simulink model "pruebaSF3_truetime"  (R2018a)
settings: Solver=FixedStepAuto  StartTime=0.0  StopTime=6  FixedStep=0.0001  RelTol=1e-3
InitFcn:
  | SimulinkInit
values from neighbouring files (symbols this model uses):
  C = C1+C2+C3+Cl    (= 0.002654)    [SimulinkInit.m]
  C3 = 610e-6    (= 0.00061)    [SimulinkInit.m]
  J = 0.3    [SimulinkInit.m]
  K1 = 1.15    [SimulinkInit.m]
  K2 = 1    [SimulinkInit.m]
  K3 = 1    [SimulinkInit.m]
  L1 = 40e-3    (= 0.04)    [SimulinkInit.m]
  L2 = 5e-3    (= 0.005)    [SimulinkInit.m]
  L3 = 30e-3    (= 0.03)    [SimulinkInit.m]
  L4 = 5.2    [SimulinkInit.m]
  P = 0.1    [SimulinkInit.m]
  R1 = 0.1    [SimulinkInit.m]
  R2 = 0.1    [SimulinkInit.m]
  R3 = 1e-3    (= 0.001)    [SimulinkInit.m]
  R4 = 10    [SimulinkInit.m]
  R5 = 10    [SimulinkInit.m]
  Tao1 = 0.5    [SimulinkInit.m]
  Tao2 = 0.125    [SimulinkInit.m]
libraries: dsparch4 x5, truetime x2, mpclib x2, simulink x1, powerlib_meascontrol x1
settings Model: Creator=carma  LastModifiedBy=carma
settings CodeAppCC: StateflowObjectComments=on
settings SimscapeCC: SimscapeNormalizeSystem=off

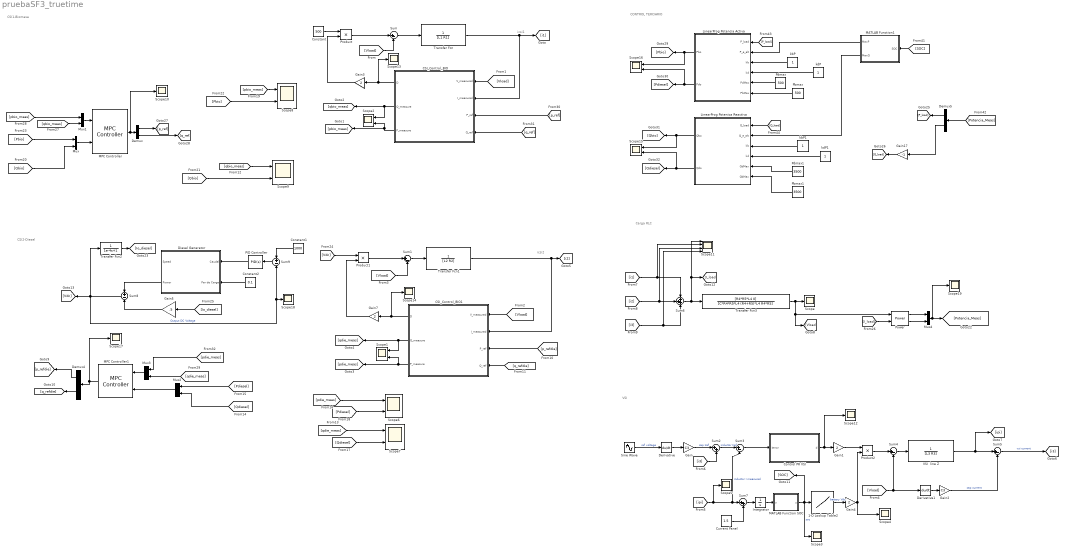
== system pruebaSF3_truetime ==
  note: Carga RLC
  note: CONTROL TERCIARIO
  note: CSI1-Biomasa
  note: CSI2-Diesel
  note: VSI
  note: icsi2
  note: icsi1
  1-D Lookup Table2 : Lookup_n-D  NumberOfTableDimensions=1  BreakpointsForDimension1=[0 10 20 30 40 50 70 80 100]  Table=[0 10 200 500 800 1000 1140 1150 1200]  InternalRulePriority=Speed  RndMeth=Simplest  InputSameDT=on
  CSI_Control_BIO : Subsystem  mask{A=[0.0201   -0.039932     0.01986], B=[1     -1.9966       0.998], T=0.0001, st_time=.1, Dn=[1     -1.0364], Dd=[1    -0.96364]}
      mask prompts: A "Numerador del control PR(z)"; B "Denominador del control PR(z)"; T "Tiempo de muestreo"; st_time "Tiempo_muerto"; Dn "Dn (Numerador de D(z))"; Dd "Dd (numerador de D(z))"
      mask DialogControl descripcion Prompt: Lazo de control de corriente para inversor monofasico. La entrada es un setpoint de potencia [P, Q]. Con ese setpoint se calcula la referencia de corriente sinusoidal deacuerdo a la tension medida de la red. Por lo anterior este controlador solo es valido para un inversor conectado a la red pues hara que se comporte como un CSI.
      mask DialogControl Control2 Prompt: Dn y Dd corresponden al numerador y denominador de la funcion de transferencia en Z (denominada D(z)) que hara un desfase de 90 de las señales medidas de tension y corriente del inversor. Estos desfases permiten mimificar las señales alfa y beta, de esta forma usar la misma teoria de potencia instantanea para el caso monofasico.
  CSI_Control_BIO1 : Subsystem  mask{A=[0.0201   -0.039932     0.01986], B=[1     -1.9966       0.998], T=0.0001, st_time=.1, Dn=[1     -1.0364], Dd=[1    -0.96364]}
      mask prompts: A "Numerador del control PR(z)"; B "Denominador del control PR(z)"; T "Tiempo de muestreo"; st_time "Tiempo_muerto"; Dn "Dn (Numerador de D(z))"; Dd "Dd (numerador de D(z))"
      mask DialogControl descripcion Prompt: Lazo de control de corriente para inversor monofasico. La entrada es un setpoint de potencia [P, Q]. Con ese setpoint se calcula la referencia de corriente sinusoidal deacuerdo a la tension medida de la red. Por lo anterior este controlador solo es valido para un inversor conectado a la red pues hara que se comporte como un CSI.
      mask DialogControl Control2 Prompt: Dn y Dd corresponden al numerador y denominador de la funcion de transferencia en Z (denominada D(z)) que hara un desfase de 90 de las señales medidas de tension y corriente del inversor. Estos desfases permiten mimificar las señales alfa y beta, de esta forma usar la misma teoria de potencia instantanea para el caso monofasico.
  Constant : Constant  Value=500
  Constant1 : Constant  Value=1000
  Constant2 : Constant  Value=0.1
  Control PR VSI : Subsystem
  Current Panel : Constant  Value=1.5
  Demux : Demux  Outputs=2
  Demux4 : Demux  Outputs=2
  Demux5 : Demux  Outputs=2
  Derivative : Derivative
  Derivative1 : Derivative
  Diesel Generator : Subsystem
  Gain : Gain  Gain=C3
  Gain{1,3..4,7} (4 alike) : Gain  Gain=2
  Gain17 : Gain  Gain=-1
  Gain2 : Gain  Gain=C3
  Gain5 : Gain  Gain=.5
  Integrator : Integrator  LimitOutput=on  UpperSaturationLimit=1  LowerSaturationLimit=0
  LinearProg Potencia Activa : MATLAB Function  TreatAsAtomicUnit=on  SystemSampleTime=.03
  LinearProg Potenica Reactiva : MATLAB Function  TreatAsAtomicUnit=on  SystemSampleTime=.03
  "MATLAB Function SOC " : MATLAB Function  TreatAsAtomicUnit=on
  MATLAB Function1 : MATLAB Function  TreatAsAtomicUnit=on
  MPC Controller : mpclib/MPC Controller  mpcobj=mpcobj  x0=[]  is_multiple=0  enable_value=0  return_u0=off  updateMPCinCallerWorkspace=on  ref_from_ws=off  ref_signal_name=[]  ref_preview=on  md_from_ws=off  md_signal_name=[]  md_preview=on  from_project=off  project_file=MPCtask.mat  md_inport=off  mv_inport=off  cost_outport=off  return_sequence=off  return_qpstatus=off  return_state=off  state_inport=off  lims_inport=off  cc_inport=off  ywt_inport=off  is_designfromscratch=0  uwt_inport=off  duwt_inport=off  rhoeps_inport=off  uref_inport=off  n_ts=0.1  n_p=100  n_mv=2  n_md=0  n_ud=0  n_mo=2  n_uo=0  BlockDataType=double  SampleTimeInherited=off  switch_inport=off
  MPC Controller1 : mpclib/MPC Controller  mpcobj=mpcobj  x0=[]  is_multiple=0  enable_value=0  return_u0=off  updateMPCinCallerWorkspace=on  ref_from_ws=off  ref_signal_name=[]  ref_preview=on  md_from_ws=off  md_signal_name=[]  md_preview=on  from_project=off  project_file=MPCtask.mat  md_inport=off  mv_inport=off  cost_outport=off  return_sequence=off  return_qpstatus=off  return_state=off  state_inport=off  lims_inport=off  cc_inport=off  ywt_inport=off  is_designfromscratch=0  uwt_inport=off  duwt_inport=off  rhoeps_inport=off  uref_inport=off  n_ts=0.1  n_p=100  n_mv=2  n_md=0  n_ud=0  n_mo=2  n_uo=0  BlockDataType=double  SampleTimeInherited=off  switch_inport=off
  Mux{,1..4} (5 alike) : Mux  Inputs=2
  PID Controller : simulink/Continuous/PID Controller  Controller=PID  TimeDomain=Continuous-time  SampleTime=-1  IntegratorMethod=Forward Euler  FilterMethod=Forward Euler  Form=Parallel  UseFilter=on  ControllerParametersSource=internal  P=0.000853612192208084  I=3.94394231511782e-05  D=0.00224356290205903  N=0.155980576752107  InitialConditionSource=internal  InitialConditionForIntegrator=0  InitialConditionForFilter=0  ExternalReset=none  LimitOutput=off  UpperSaturationLimit=inf  LowerSaturationLimit=-inf  LinearizeAsGain=on  AntiWindupMode=none  Kb=1  TrackingMode=off  Kt=1  PParamMin=[]  PParamMax=[]  IParamMin=[]  IParamMax=[]  DParamMin=[]  DParamMax=[]  NParamMin=[]  NParamMax=[]  KbParamMin=[]  KbParamMax=[]  KtParamMin=[]  KtParamMax=[]  POutMin=[]  POutMax=[]  IOutMin=[]  IOutMax=[]  DOutMin=[]  DOutMax=[]  NOutMin=[]  NOutMax=[]  KbOutMin=[]  KbOutMax=[]  KtOutMin=[]  KtOutMax=[]  IntegratorOutMin=[]  IntegratorOutMax=[]  FilterOutMin=[]  FilterOutMax=[]  SumOutMin=[]  SumOutMax=[]  SumI1OutMin=[]  SumI1OutMax=[]  SumI2OutMin=[]  SumI2OutMax=[]  SumI3OutMin=[]  SumI3OutMax=[]  SumDOutMin=[]  SumDOutMax=[]  SaturationOutMin=[]  SaturationOutMax=[]  IntegratorContinuousStateAttributes=''  IntegratorStateMustResolveToSignalObject=off  IntegratorRTWStateStorageClass=Auto  FilterContinuousStateAttributes=''  FilterStateMustResolveToSignalObject=off  FilterRTWStateStorageClass=Auto  DifferentiatorICPrevScaledInput=0  DifferentiatorOutMin=[]  DifferentiatorOutMax=[]  InitialConditionSetting=State (most efficient)  FilterDiffOutCoefMin=[]  FilterDiffOutCoefMax=[]  SumDenOutMin=[]  SumDenOutMax=[]  SumNumOutMin=[]  SumNumOutMax=[]  ReciprocalOutMin=[]  ReciprocalOutMax=[]  DivideOutMin=[]  DivideOutMax=[]  TunerSelectOption=Transfer Function Based (PID Tuner App)
  Pbmax : Constant  Value=500
  Pbmax1 : Constant  Value=3500
  Pdmax : Constant  Value=500
  Pdmax1 : Constant  Value=3500
  Power : powerlib_meascontrol/Measurements/Power  Freq=60  Vinit=[1, 0]  Iinit=[1, 0]  Ts=0
      settings: SourceProductName=Simscape Power Systems
  Product : Product
  Product1 : Product
  Product2 : Product
  Scope{,3..5,10,12..14,17..19} (11 alike) : Scope
  Scope{1..2,6..9,15..16} (8 alike) : Scope  NumInputPorts=2
  Scope11 : Scope  NumInputPorts=4
  Sine Wave : Sin  Amplitude=170  Frequency=2*pi*60  SampleTime=0
  Sum{,1,3..5} (5 alike) : Sum  Inputs=|+-
  Sum2 : Sum  Inputs=|++
  Sum6 : Sum  Inputs=3
  Sum7 : Sum  Inputs=|++
  Sum8 : Sum  Inputs=+-
  Sum9 : Sum  Inputs=+-
  Transfer Fcn : TransferFcn  Denominator=[L1 R1]
  Transfer Fcn1 : TransferFcn  Denominator=[L2 R2]
  Transfer Fcn2 : TransferFcn  Denominator=[1e-4 1]
  Transfer Fcn3 : TransferFcn  Numerator=[R4*R5*L4 0]  Denominator=[C*R4*R5*L4 (R4+R5)*L4 R4*R5]
  VSI  line Z : TransferFcn  Denominator=[L3 R3]
  kbP : Constant
  kbP1 : Constant
  kdP : Constant
  kdP1 : Constant
  wires:
  Sum/1 -> Transfer Fcn/1
  [Vload] -> Sum/2
  Product/1 -> Sum/1
  Constant/1 -> Product/1
  Gain3/1 -> Product/2
  CSI_Control_BIO/2(Q_measure) -> [qbio_meas], Scope2/1
  Transfer Fcn/1 -> [i1], CSI_Control_BIO/2(I_measured)
  [Vload] -> CSI_Control_BIO/1(V_measured)
  CSI_Control_BIO/1(D) -> Scope13/1, Gain3/1
  Gain7/1 -> Product1/2
  CSI_Control_BIO1/1(D) -> Scope14/1, Gain7/1
  Transfer Fcn1/1 -> [i2], CSI_Control_BIO1/2(I_measured)
  [Vload] -> CSI_Control_BIO1/1(V_measured)
  CSI_Control_BIO1/3(P_measure) -> Scope1/2, [pdie_meas]
  CSI_Control_BIO1/2(Q_measure) -> [qdie_meas], Scope1/1
  Product1/1 -> Sum1/1
  [Vdc] -> Product1/1
  Sum1/1 -> Transfer Fcn1/1
  [Vload] -> Sum1/2
  Sine Wave/1 -> Derivative/1  "ref voltage"
  Derivative/1 -> Gain/1
  Gain/1 -> Sum2/1  "cap Iref"
  Sum2/1 -> Sum3/1  "inductor Iref"
  Sum3/1 -> Control PR VSI/1(Ierror)
  Control PR VSI/1(d) -> Scope12/1, Gain1/1
  Gain1/1 -> Product2/1
  Product2/1 -> Sum4/1
  [Vload] -> Sum4/2, Derivative1/1
  Derivative1/1 -> Gain2/1
  Sum4/1 -> VSI  line Z/1
  VSI  line Z/1 -> [ipi], Sum5/1
  Gain2/1 -> Sum5/2  "cap current"
  Sum5/1 -> [i3]  "vsi current"
  [ipi] -> Scope5/1, Sum7/1, Sum3/2  "inductor I measured"
  [i3] -> Sum2/2
  Integrator/1 -> "MATLAB Function SOC "/1(u)
  "MATLAB Function SOC "/1(y) -> [SOC], Scope3/1, 1-D Lookup Table2/1  "soc"
  1-D Lookup Table2/1 -> Gain4/1  "battery Vdc"
  [i1] -> Scope11/2, Sum6/1
  [i2] -> Scope11/3, Sum6/2
  [i3] -> Sum6/3, Scope11/4
  Sum6/1 -> [I_load], Scope11/1, Transfer Fcn3/1
  [qdie_meas] -> Scope7/1
  Mux3/1 -> MPC Controller1/1
  [pdie_meas] -> Mux3/1
  Demux4/2 -> [q_refdie]
  Mux2/1 -> MPC Controller1/2
  [qdie_meas] -> Mux3/2
  [Qdiesel] -> Scope7/2
  MPC Controller1/1 -> Demux4/1, Scope17/1
  [Pdiesel] -> Scope6/2
  [pdie_meas] -> Scope6/1
  Demux4/1 -> [p_refdie]
  [pbio_meas] -> Mux1/1
  [Pbio] -> Scope8/2
  [qbio_meas] -> Scope9/1
  [qbio_meas] -> Mux1/2
  MPC Controller/1 -> Scope10/1, Demux/1
  [Qbio] -> Scope9/2
  Mux1/1 -> MPC Controller/1
  Demux/2 -> [q_ref]
  [pbio_meas] -> Scope8/1
  Mux/1 -> MPC Controller/2
  Demux/1 -> [p_ref]
  [SOC] -> MATLAB Function1/1(SOC)
  kdP/1 -> LinearProg Potencia Activa/4(kd)
  Pdmax/1 -> LinearProg Potencia Activa/5(PdMax)
  Gain17/1 -> [Q_load]
  kbP1/1 -> LinearProg Potenica Reactiva/3(kb)
  LinearProg Potencia Activa/2(Pdo) -> Scope16/2, [Pdiesel]
  [P_load] -> LinearProg Potencia Activa/1(P_load)
  kbP/1 -> LinearProg Potencia Activa/3(kb)
  Pbmax/1 -> LinearProg Potencia Activa/6(PbMax)
  MATLAB Function1/2(MaxQ) -> LinearProg Potenica Reactiva/2(Q_e_alt)
  MATLAB Function1/1(MaxP) -> LinearProg Potencia Activa/2(P_e_alt)
  kdP1/1 -> LinearProg Potenica Reactiva/4(kd)
  LinearProg Potencia Activa/1(Pbo) -> Scope16/1, [Pbio]
  Demux5/1 -> [P_load]
  [Potencia_Meas] -> Demux5/1
  Demux5/2 -> Gain17/1
  Pbmax1/1 -> LinearProg Potenica Reactiva/6(QbMax)
  Pdmax1/1 -> LinearProg Potenica Reactiva/5(QdMax)
  LinearProg Potenica Reactiva/1(Qbo) -> Scope15/1, [Qbio]
  LinearProg Potenica Reactiva/2(Qdo) -> Scope15/2, [Qdiesel]
  [Q_load] -> LinearProg Potenica Reactiva/1(Q_load)
  Power/1 -> Mux4/1
  [I_load] -> Power/2
  Power/2 -> Mux4/2
  Mux4/1 -> Scope19/1, [Potencia_Meas]
  Transfer Fcn3/1 -> Power/1, [Vload], Scope/1
  Gain4/1 -> Product2/2, Scope4/1
  [p_refdie] -> CSI_Control_BIO1/3(P_ref)
  [q_refdie] -> CSI_Control_BIO1/4(Q_ref)
  [Pdiesel] -> Mux2/1
  [Pbio] -> Mux/1
  [Qbio] -> Mux/2
  [Qdiesel] -> Mux2/2
  CSI_Control_BIO/3(P_measure) -> [pbio_meas], Scope2/2
  [p_ref] -> CSI_Control_BIO/3(P_ref)
  [q_ref] -> CSI_Control_BIO/4(Q_ref)
  Sum7/1 -> Integrator/1
  Current Panel/1 -> Sum7/2
  [Io_diesel] -> Gain5/1
  Constant1/1 -> Sum9/1
  Transfer Fcn2/1 -> [Io_diesel]
  Diesel Generator/2(Power) -> Sum8/1
  Gain5/1 -> Sum8/2
  Constant2/1 -> Diesel Generator/2(Par de Carga)
  PID Controller/1 -> Diesel Generator/1(Caudal)
  Sum8/1 -> [Vdc], Scope18/1, Sum9/2, Transfer Fcn2/1  "Output DC Voltage"
  Sum9/1 -> PID Controller/1

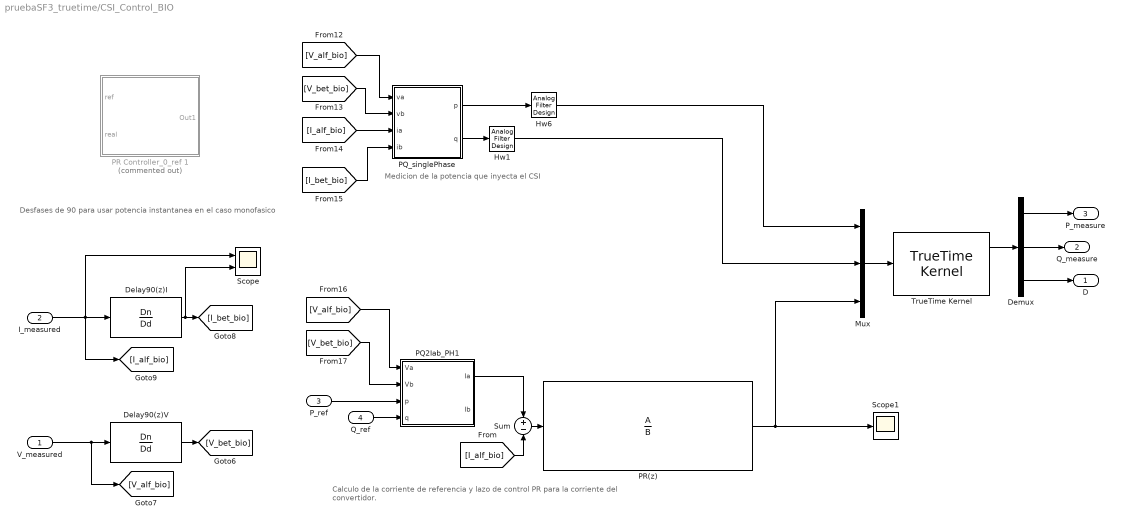
== system pruebaSF3_truetime/CSI_Control_BIO ==
  note: Medicion de la potencia que inyecta el CSI
  note: Desfases de 90 para usar potencia
      | instantanea en el caso monofasico
  note: Calculo de la corriente de referencia
      | y lazo de control PR para la corriente
      | del convertidor.
  V_measured : Inport
  I_measured : Inport  Port=2
  P_ref : Inport  Port=3
  Q_ref : Inport  Port=4
  Delay90(z)I : DiscreteTransferFcn  Numerator=Dn  Denominator=Dd  SampleTime=T
  Delay90(z)V : DiscreteTransferFcn  Numerator=Dn  Denominator=Dd  SampleTime=T
  Demux : Demux  Outputs=3
  Hw1 : dsparch4/Analog Filter Design  method=Bessel  filttype=Lowpass  N=4  Wlo=30*2*pi  Whi=80  Rp=2  Rs=80
  Hw6 : dsparch4/Analog Filter Design  method=Bessel  filttype=Lowpass  N=4  Wlo=30*2*pi  Whi=80  Rp=2  Rs=80
  Mux : Mux  Inputs=3
  PQ2Iab_PH1 : MATLAB Function  TreatAsAtomicUnit=on
  PQ_singlePhase : MATLAB Function  TreatAsAtomicUnit=on
  PR Controller_0_ref 1 : Subsystem  Commented=on  mask{Kp=40/100, Ki=200, wa=2, w0=60*2*pi, st_time=1e-3}
      mask prompts: Kp "Ganancia Proporcional"; Ki "Ganancia Integral"; wa "Ancho camapana resonancia"; w0 "Frecuencia Central"; st_time "Tiempo muerto (Start)"
      mask Display:
      | port_label('input',1,'ref')
      | port_label('input',2,'sens')
      | port_label('output',1,'out')
      | 
      | plot(.4+[0:.01:pi/10], .32+sin(40*[0:.01:pi/10])/13)
      | 
      | plot([.4 .6],.05+[.5 .7])
      | plot([.4 .6],.05+[.9 .7])
      | plot([.4 .4],.05+[.9 .5])
      | 
      | text(.27,.37,'\fontsize{25} \int', 'texmode', 'on')
  PR(z) : DiscreteTransferFcn  Numerator=A  Denominator=B  SampleTime=T
  Scope : Scope  NumInputPorts=2
  Scope1 : Scope
  Sum : Sum  Inputs=+-
  TrueTime Kernel : truetime/TrueTime Kernel  sfun=BIO_init  args=[]  ninputsoutputs=[3 3]  ntriggers=0  trigtype=falling  nwnodenbr=[]  clockoffsetdrift=[0 0]  schedoutput=on  battery=off  poweroutput=off
  D : Outport
  Q_measure : Outport  Port=2
  P_measure : Outport  Port=3
  wires:
  I_measured/1 -> Scope/1, Delay90(z)I/1, [I_alf_bio]
  PQ_singlePhase/2(q) -> Hw1/1
  [V_bet_bio] -> PQ2Iab_PH1/2(Vb)
  Delay90(z)I/1 -> Scope/2, [I_bet_bio]
  [I_bet_bio] -> PQ_singlePhase/4(ib)
  [I_alf_bio] -> PQ_singlePhase/3(ia)
  [V_alf_bio] -> PQ2Iab_PH1/1(Va)
  PQ_singlePhase/1(p) -> Hw6/1
  Delay90(z)V/1 -> [V_bet_bio]
  [V_bet_bio] -> PQ_singlePhase/2(vb)
  [V_alf_bio] -> PQ_singlePhase/1(va)
  V_measured/1 -> Delay90(z)V/1, [V_alf_bio]
  P_ref/1 -> PQ2Iab_PH1/3(p)
  Q_ref/1 -> PQ2Iab_PH1/4(q)
  Sum/1 -> PR(z)/1
  [I_alf_bio] -> Sum/2
  PQ2Iab_PH1/1(Ia) -> Sum/1
  PR(z)/1 -> Scope1/1, Mux/3
  Hw6/1 -> Mux/1
  Hw1/1 -> Mux/2
  Mux/1 -> TrueTime Kernel/1
  TrueTime Kernel/1 -> Demux/1
  Demux/3 -> D/1
  Demux/1 -> P_measure/1
  Demux/2 -> Q_measure/1

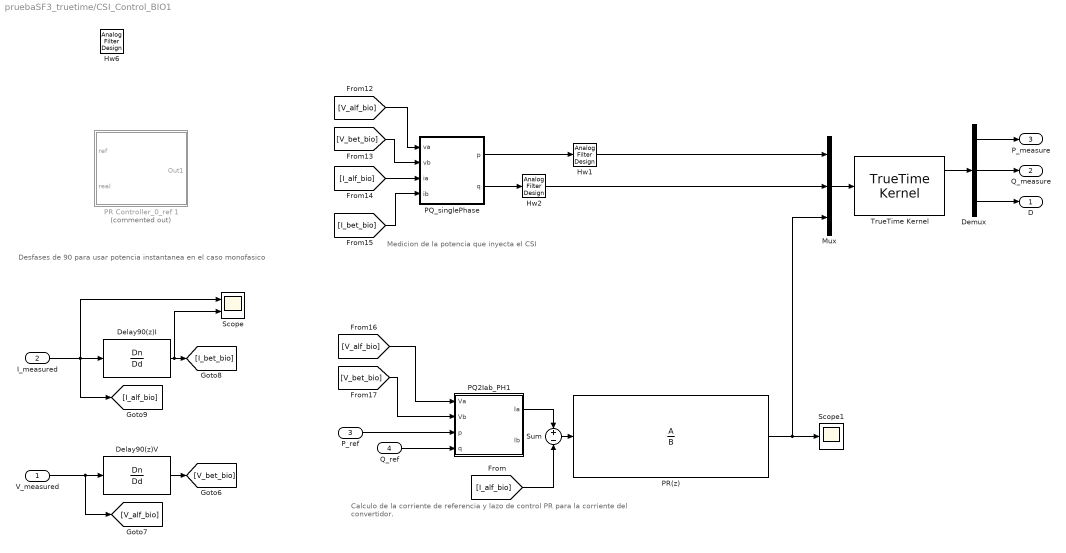
== system pruebaSF3_truetime/CSI_Control_BIO1 ==
  note: Medicion de la potencia que inyecta el CSI
  note: Desfases de 90 para usar potencia
      | instantanea en el caso monofasico
  note: Calculo de la corriente de referencia
      | y lazo de control PR para la corriente
      | del convertidor.
  V_measured : Inport
  I_measured : Inport  Port=2
  P_ref : Inport  Port=3
  Q_ref : Inport  Port=4
  Delay90(z)I : DiscreteTransferFcn  Numerator=Dn  Denominator=Dd  SampleTime=T
  Delay90(z)V : DiscreteTransferFcn  Numerator=Dn  Denominator=Dd  SampleTime=T
  Demux : Demux  Outputs=3
  Hw1 : dsparch4/Analog Filter Design  method=Bessel  filttype=Lowpass  N=4  Wlo=30*2*pi  Whi=80  Rp=2  Rs=80
  Hw2 : dsparch4/Analog Filter Design  method=Bessel  filttype=Lowpass  N=4  Wlo=30*2*pi  Whi=80  Rp=2  Rs=80
  Hw6 : dsparch4/Analog Filter Design  method=Bessel  filttype=Lowpass  N=4  Wlo=30*2*pi  Whi=80  Rp=2  Rs=80
  Mux : Mux  Inputs=3
  PQ2Iab_PH1 : MATLAB Function  TreatAsAtomicUnit=on
  PQ_singlePhase : MATLAB Function  TreatAsAtomicUnit=on
  PR Controller_0_ref 1 : Subsystem  Commented=on  mask{Kp=40/100, Ki=200, wa=2, w0=60*2*pi, st_time=1e-3}
      mask prompts: Kp "Ganancia Proporcional"; Ki "Ganancia Integral"; wa "Ancho camapana resonancia"; w0 "Frecuencia Central"; st_time "Tiempo muerto (Start)"
      mask Display:
      | port_label('input',1,'ref')
      | port_label('input',2,'sens')
      | port_label('output',1,'out')
      | 
      | plot(.4+[0:.01:pi/10], .32+sin(40*[0:.01:pi/10])/13)
      | 
      | plot([.4 .6],.05+[.5 .7])
      | plot([.4 .6],.05+[.9 .7])
      | plot([.4 .4],.05+[.9 .5])
      | 
      | text(.27,.37,'\fontsize{25} \int', 'texmode', 'on')
  PR(z) : DiscreteTransferFcn  Numerator=A  Denominator=B  SampleTime=T
  Scope : Scope  NumInputPorts=2
  Scope1 : Scope
  Sum : Sum  Inputs=+-
  TrueTime Kernel : truetime/TrueTime Kernel  sfun=DIESEL_init  args=[]  ninputsoutputs=[3 3]  ntriggers=0  trigtype=falling  nwnodenbr=[]  clockoffsetdrift=[0 0]  schedoutput=on  battery=off  poweroutput=off
  D : Outport
  Q_measure : Outport  Port=2
  P_measure : Outport  Port=3
  wires:
  I_measured/1 -> Scope/1, Delay90(z)I/1, [I_alf_bio]
  PQ_singlePhase/2(q) -> Hw2/1
  [V_bet_bio] -> PQ2Iab_PH1/2(Vb)
  Delay90(z)I/1 -> Scope/2, [I_bet_bio]
  [I_bet_bio] -> PQ_singlePhase/4(ib)
  [I_alf_bio] -> PQ_singlePhase/3(ia)
  [V_alf_bio] -> PQ2Iab_PH1/1(Va)
  Delay90(z)V/1 -> [V_bet_bio]
  [V_bet_bio] -> PQ_singlePhase/2(vb)
  [V_alf_bio] -> PQ_singlePhase/1(va)
  V_measured/1 -> Delay90(z)V/1, [V_alf_bio]
  P_ref/1 -> PQ2Iab_PH1/3(p)
  Q_ref/1 -> PQ2Iab_PH1/4(q)
  Sum/1 -> PR(z)/1
  [I_alf_bio] -> Sum/2
  PQ2Iab_PH1/1(Ia) -> Sum/1
  Demux/3 -> D/1
  Demux/2 -> Q_measure/1
  Mux/1 -> TrueTime Kernel/1
  TrueTime Kernel/1 -> Demux/1
  PR(z)/1 -> Mux/3, Scope1/1
  PQ_singlePhase/1(p) -> Hw1/1
  Demux/1 -> P_measure/1
  Hw2/1 -> Mux/2
  Hw1/1 -> Mux/1

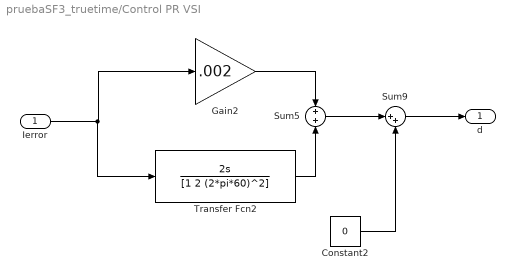
== system pruebaSF3_truetime/Control PR VSI ==
  Ierror : Inport
  Constant2 : Constant  Value=0
  Gain2 : Gain  Gain=.002
  Sum5 : Sum  Inputs=+|+
  Sum9 : Sum  Inputs=|++
  Transfer Fcn2 : TransferFcn  Numerator=[2 0]  Denominator=[1 2 (2*pi*60)^2]
  d : Outport
  wires:
  Constant2/1 -> Sum9/2
  Sum5/1 -> Sum9/1
  Transfer Fcn2/1 -> Sum5/2
  Gain2/1 -> Sum5/1
  Ierror/1 -> Transfer Fcn2/1, Gain2/1
  Sum9/1 -> d/1

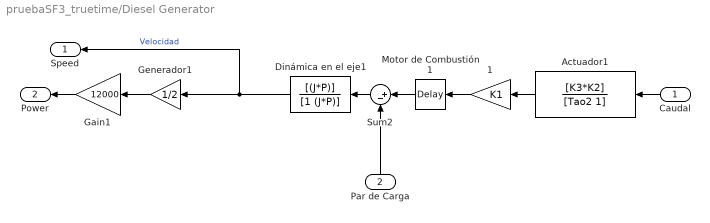
== system pruebaSF3_truetime/Diesel Generator ==
  Caudal : Inport
  Par de Carga : Inport  Port=2
  " 1" : Gain  Gain=K1
  " Generador1" : Gain  Gain=1/2
  Actuador1 : TransferFcn  Numerator=[K3*K2]  Denominator=[Tao2 1]
  Dinámica en el eje1 : TransferFcn  Numerator=[(J*P)]  Denominator=[1 (J*P)]
  Gain1 : Gain  Gain=12000
  Motor de Combustión1 : TransportDelay  DelayTime=Tao1
  Sum2 : Sum  Inputs=|+-
  Speed : Outport
  Power : Outport  Port=2
  wires:
  " 1"/1 -> Motor de Combustión1/1
  " Generador1"/1 -> Gain1/1
  Motor de Combustión1/1 -> Sum2/1
  Actuador1/1 -> " 1"/1
  Dinámica en el eje1/1 -> Speed/1, " Generador1"/1  "Velocidad"
  Sum2/1 -> Dinámica en el eje1/1
  Caudal/1 -> Actuador1/1
  Par de Carga/1 -> Sum2/2
  Gain1/1 -> Power/1

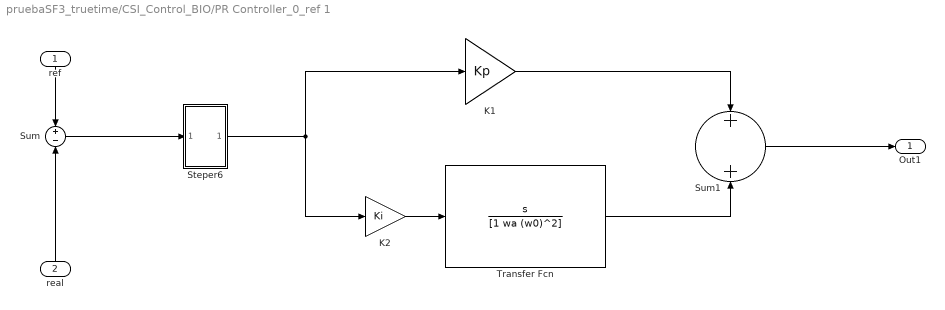
== system pruebaSF3_truetime/CSI_Control_BIO/PR Controller_0_ref 1 ==
  ref : Inport
  real : Inport  Port=2
  K1 : Gain  Gain=Kp
  K2 : Gain  Gain=Ki
  Steper6 : Subsystem
  Sum : Sum  Inputs=+-
  Sum1 : Sum  Inputs=+|+
  Transfer Fcn : TransferFcn  Numerator=[1 0]  Denominator=[1 wa (w0)^2]
  Out1 : Outport
  wires:
  real/1 -> Sum/2
  ref/1 -> Sum/1
  Sum/1 -> Steper6/1(In1)
  K1/1 -> Sum1/1
  Transfer Fcn/1 -> Sum1/2
  K2/1 -> Transfer Fcn/1
  Steper6/1(Out1) -> K1/1, K2/1
  Sum1/1 -> Out1/1

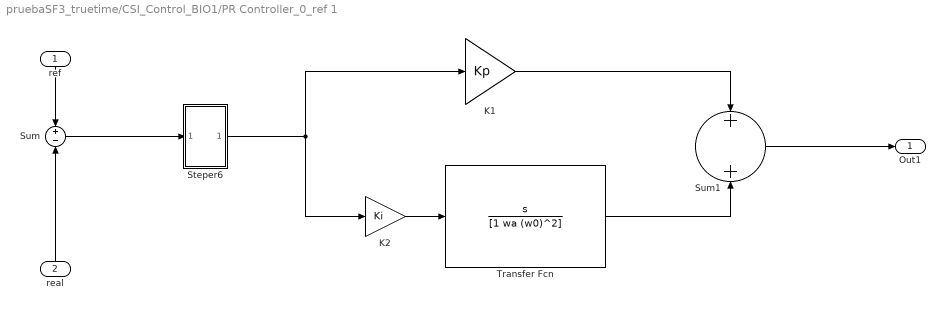
== system pruebaSF3_truetime/CSI_Control_BIO1/PR Controller_0_ref 1 ==
  ref : Inport
  real : Inport  Port=2
  K1 : Gain  Gain=Kp
  K2 : Gain  Gain=Ki
  Steper6 : Subsystem
  Sum : Sum  Inputs=+-
  Sum1 : Sum  Inputs=+|+
  Transfer Fcn : TransferFcn  Numerator=[1 0]  Denominator=[1 wa (w0)^2]
  Out1 : Outport
  wires:
  real/1 -> Sum/2
  ref/1 -> Sum/1
  Sum/1 -> Steper6/1(In1)
  K1/1 -> Sum1/1
  Transfer Fcn/1 -> Sum1/2
  K2/1 -> Transfer Fcn/1
  Steper6/1(Out1) -> K1/1, K2/1
  Sum1/1 -> Out1/1

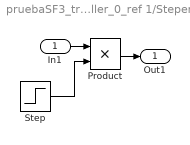
== system pruebaSF3_truetime/CSI_Control_BIO/PR Controller_0_ref 1/Steper6 ==
  In1 : Inport
  Product : Product
  Step : Step  Time=st_time  SampleTime=0
  Out1 : Outport
  wires:
  Product/1 -> Out1/1
  In1/1 -> Product/1
  Step/1 -> Product/2

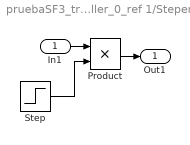
== system pruebaSF3_truetime/CSI_Control_BIO1/PR Controller_0_ref 1/Steper6 ==
  In1 : Inport
  Product : Product
  Step : Step  Time=st_time  SampleTime=0
  Out1 : Outport
  wires:
  Product/1 -> Out1/1
  In1/1 -> Product/1
  Step/1 -> Product/2

== matlab function pruebaSF3_truetime/CSI_Control_BIO1/PQ2Iab_PH1 ==
  data: Va input; Ia output; Vb input; p input; q input; Ib output
function [Ia, Ib] = fcn(Va, Vb, p, q)
%#codegen

% divide by zero protection
if(abs((Va^2+Vb^2))<=1000*eps(0))
    det = 1/eps(0);
else
    det = 1/(Va^2+Vb^2); % constante auxiliar
end;
%det = 1/(Va^2+Vb^2);

Mat = det*[Va Vb; Vb -Va];
Iab = Mat*[2*p;2*q];

Iaaux = Iab(1);
Ibaux = Iab(2);

ilim=1e3;

if(Iaaux>ilim)
    Iaaux=ilim;
end;
if(Iaaux<-ilim)
    Iaaux =-ilim;    
end;

if(isnan(Iaaux))
    Iaaux=0;
end;
%-----------------


if(Ibaux>ilim)
    Ibaux=ilim;
end;
if(Ibaux<-ilim)
    Ibaux =-ilim;    
end;

if(isnan(Ibaux))
    Ibaux=0;
end;
%-----------------


Ia = Iaaux;
Ib = Ibaux;

== matlab function pruebaSF3_truetime/CSI_Control_BIO1/PQ_singlePhase ==
  data: va input; p output; vb input; ia input; ib input; q output
function [p, q] = fcn(va, vb, ia, ib)
% Esta funcion calcula la potencia activa y reactiva instantanea
% para el caso mnosofasico. En la revision de 2 papers he observado
% que una manera de extender la teoria de potencia al caso monofasico
% es asumiendo la tension o corriente de una fase como la componente
% alpha y hacer un desfase de 90 grados para obtener una version
% artificial de beta.

paux=va*ia+vb*ib;
if(paux > 20e4)
    paux = 20e4;
end
if(paux < -20e4)
    paux = -20e-4;
end

p = paux/2; % potencia activa instantanea

qaux = vb*ia-va*ib;

if(qaux>20e4)
    qaux=20e4;
end
if(qaux<-20e4)
    qaux=-20e4;
end

q = qaux/2; % potencia reactiva instantanea

== matlab function pruebaSF3_truetime/CSI_Control_BIO/PQ_singlePhase ==
  data: va input; p output; vb input; ia input; ib input; q output
function [p, q] = fcn(va, vb, ia, ib)
% Esta funcion calcula la potencia activa y reactiva instantanea
% para el caso mnosofasico. En la revision de 2 papers he observado
% que una manera de extender la teoria de potencia al caso monofasico
% es asumiendo la tension o corriente de una fase como la componente
% alpha y hacer un desfase de 90 grados para obtener una version
% artificial de beta.

paux=va*ia+vb*ib;
if(paux > 20e4)
    paux = 20e4;
end
if(paux < -20e4)
    paux = -20e-4;
end

p = paux/2; % potencia activa instantanea

qaux = vb*ia-va*ib;

if(qaux>20e4)
    qaux=20e4;
end
if(qaux<-20e4)
    qaux=-20e4;
end

q = qaux/2; % potencia reactiva instantanea

== matlab function pruebaSF3_truetime/MATLAB Function SOC  ==
  data: u input; y output
function y = fcn(u)

y = -0.03536*u+100;

== matlab function pruebaSF3_truetime/CSI_Control_BIO/PQ2Iab_PH1 ==
  data: Va input; Ia output; Vb input; p input; q input; Ib output
function [Ia, Ib] = fcn(Va, Vb, p, q)
%#codegen

% divide by zero protection
if(abs((Va^2+Vb^2))<=1000*eps(0))
    det = 1/eps(0);
else
    det = 1/(Va^2+Vb^2); % constante auxiliar
end;
%det = 1/(Va^2+Vb^2);

Mat = det*[Va Vb; Vb -Va];
Iab = Mat*[2*p;2*q];

Iaaux = Iab(1);
Ibaux = Iab(2);

ilim=1e3;

if(Iaaux>ilim)
    Iaaux=ilim;
end;
if(Iaaux<-ilim)
    Iaaux =-ilim;    
end;

if(isnan(Iaaux))
    Iaaux=0;
end;
%-----------------


if(Ibaux>ilim)
    Ibaux=ilim;
end;
if(Ibaux<-ilim)
    Ibaux =-ilim;    
end;

if(isnan(Ibaux))
    Ibaux=0;
end;
%-----------------


Ia = Iaaux;
Ib = Ibaux;

== matlab function pruebaSF3_truetime/LinearProg Potencia Activa ==
  data: P_load input; Pbo output; P_e_alt input; kb input; kd input; PdMax input; PbMax input; Pdo output
function [Pbo, Pdo] = fcn(P_load, P_e_alt, kb, kd, PdMax, PbMax)%, P_e_alt_min)

% P_load es la potencia que se requiere en la carga.

% P_e_alt es la potencia estimada de generacion de las energias
% alternativas

% kb y kd son los pesos de las funcion de costo.

% las salidas son las potencias optimas para bio y diesel

Pb=0;
Pd=0;

D_P_e_alt = P_e_alt %- P_e_alt_min % superaavit de energia alternativa.

flagDelt = 0;

if(D_P_e_alt >= P_load)
    flagDelt = 1;
end
   

if(flagDelt==0)
    P_trad = P_load - D_P_e_alt;
    % flag: variable que indica si tiene sentido evaluar los
    % if's que se encuentran mas adelante. es decir, si flag = 0 
    % despues del primer if entonces NO se le esta pidiendo al sistema
    % mas potencia de la que puede generar y portante el problema de 
    % optimizacion lineal tiene sentido.
    % entonces 
    flag=0;

    if(P_trad>PdMax+PbMax)
        Pd=PdMax;
        Pb=PbMax;
        flag=1;
    end

    % si ambas energias tienen el mismo factor de costo.
    if(kd==kb && flag==0)
        Pb=P_trad/2;
        Pd=P_trad/2;
    end

    % si la energia diesel es mas cara que la biomasa.
    if(kd>kb && flag==0)
        if(P_trad<=PbMax)
            Pb=P_trad;
            Pd=0;
        else
            Pb=PbMax;
            Pd=P_trad-PbMax;
        end
    end

    % si la biomasa es mas cara que la diesel.
    if(kd<kb && flag==0)
        if(P_trad<=PdMax)
            Pd=P_trad;
            Pb=0;
        else
            Pd=PdMax;
            Pb=P_trad-PdMax;
        end
    end
end

Pbo=Pb;
Pdo=Pd;

== matlab function pruebaSF3_truetime/LinearProg Potenica Reactiva ==
  data: Q_load input; Qbo output; Q_e_alt input; kb input; kd input; QdMax input; QbMax input; Qdo output
function [Qbo, Qdo] = fcn(Q_load, Q_e_alt, kb, kd, QdMax, QbMax)

% Q_load es la potencia que se requiere en la carga.

% Q_e_alt es la potencia estimada de generacion de las energias
% alternativas

% kb y kd son los pesos de las funcion de costo.

% las salidas son las potencias optimas para bio y diesel

Qb=0;
Qd=0;

D_P_e_alt = Q_e_alt ;%- Q_e_alt_min % superaavit de energia alternativa.

flagDelt = 0;

if(D_P_e_alt >= Q_load)
    flagDelt = 1;
end
   

if(flagDelt==0)
    Q_trad = Q_load - D_P_e_alt;
    % flag: variable que indica si tiene sentido evaluar los
    % if's que se encuentran mas adelante. es decir, si flag = 0 
    % despues del primer if entonces NO se le esta pidiendo al sistema
    % mas potencia de la que puede generar y portante el problema de 
    % optimizacion lineal tiene sentido.
    % entonces 
    flag=0;

    if(Q_trad>QdMax+QbMax)
        Qd=QdMax;
        Qb=QbMax;
        flag=1;
    end

    % si ambas energias tienen el mismo factor de costo.
    if(kd==kb && flag==0)
        Qb=Q_trad/2;
        Qd=Q_trad/2;
    end

    % si la energia diesel es mas cara que la biomasa.
    if(kd>kb && flag==0)
        if(Q_trad<=QbMax)
            Qb=Q_trad;
            Qd=0;
        else
            Qb=QbMax;
            Qd=Q_trad-QbMax;
        end
    end

    % si la biomasa es mas cara que la diesel.
    if(kd<kb && flag==0)
        if(Q_trad<=QdMax)
            Qd=Q_trad;
            Qb=0;
        else
            Qd=QdMax;
            Qb=Q_trad-QdMax;
        end
    end
end

Qbo=Qb;
Qdo=Qd;

== matlab function pruebaSF3_truetime/MATLAB Function1 ==
  data: SOC input; MaxP output; MaxQ output
function [MaxP, MaxQ] = fcn(SOC)


%  funcion que calcula la potencia maxima que puede suministrar las fuentes
%  renovables deacuerdo a la cantidad de carga que hay almancenada en la
%  bateria. esta va de 0 a 100%


% estoc valores que aparecen a continuacion se pusieron de manera
% arbitraria. corresponde a una persona con especialidad en la parte de
% potencia electrica determinar el verdadero algoritmo para hallar la
% potencia que deberia suministrar el nodo de energia renovable deacuerdo a
% la carga de la bateria.

MaxP = 0;
MaxQ = 0;

if( SOC >= 90 )
    MaxP = 500;
    MaxQ = 5000;
end

if( SOC <= 90 )
    MaxP = 200;
    MaxQ = 4000;
end

if( SOC <= 70 )
    MaxP = 100;
    MaxQ = 1000;
end

if( SOC <= 60 )
    MaxP = 50;
    MaxQ = 500;
end
